simulink model "simple_RRR_l5controller"  (R2020a)
settings: Solver=ode3  StartTime=0.0  StopTime=2.1  RelTol=1e-3
libraries: roblocks x3
settings Model: Creator=yrza  LastModifiedBy=angelina

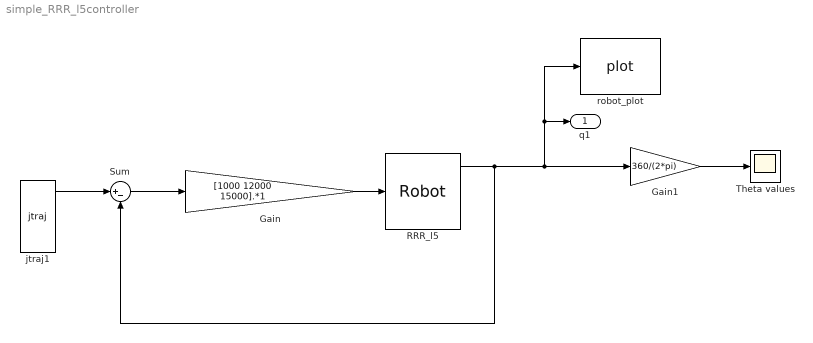
== system simple_RRR_l5controller ==
  Gain : Gain  Gain=[1000 12000 15000].*1
  Gain1 : Gain  Gain=360/(2*pi)
  RRR_l5 : roblocks/Arm/Robot  robot=RRR_l5  q0=[0 0 0]
  Sum : Sum  Inputs=|+-
  Theta values : Scope
  jtraj1 : roblocks/Toolbox/jtraj  q0=[0 0 0]  qf=[pi/2 -pi/4 -pi/4]  tmax=2  ts=0.02
  robot_plot : roblocks/Arm/plot  robot=RRR_l5  fps=10  holdplot=on
  q1 : Outport
  wires:
  RRR_l5/1 -> robot_plot/1, q1/1, Gain1/1, Sum/2
  Gain1/1 -> Theta values/1
  Sum/1 -> Gain/1
  jtraj1/1 -> Sum/1
  Gain/1 -> RRR_l5/1
